simulink model "rc_servo_sl"  (R2023a)
settings: Solver=VariableStepAuto  StartTime=0.0  StopTime=10.0  RelTol=1e-3
libraries: arduino_io_lib x3
settings Model: Creator=user  LastModifiedBy=user

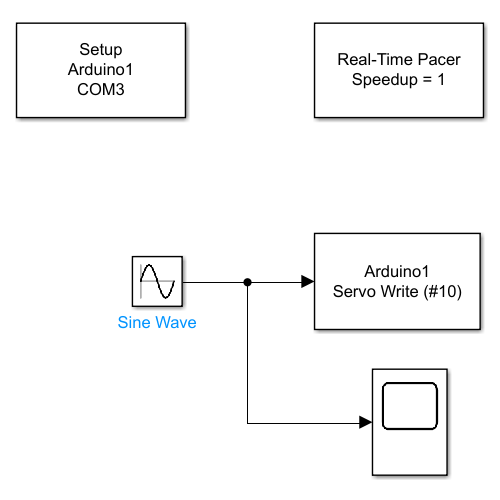
[thumbnail: Simulink's stored preview of the top-level diagram]
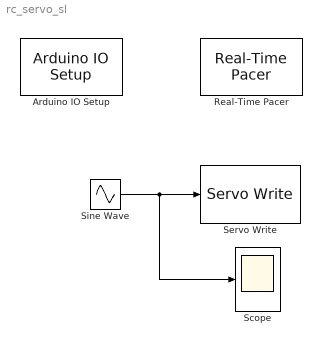
== system rc_servo_sl ==
  Arduino IO Setup : arduino_io_lib/Arduino IO Setup  Priority=3  arduinoVar=Temporary arduino variable: Arduino1  workspaceVarName=a  comPort=COM3
      settings: SourceProductName=Arduino IO Library
  Real-Time Pacer : arduino_io_lib/Real-Time Pacer  simTimePerRealTime=1
      settings: SourceProductName=Arduino IO Library
  Scope : Scope
  Servo Write : arduino_io_lib/Servo Write  arduinoVar=Temporary arduino variable: Arduino1  pinNum=10  T=0.2
      settings: SourceProductName=Arduino IO Library
  Sine Wave : Sin  Amplitude=45  Bias=90  Frequency=2  Samples=100  SampleTime=0
  wires:
  Sine Wave/1 -> Scope/1, Servo Write/1
